simulink model "mdl_sensor_imu_16b"  (R2016b)
settings: Solver=ode4  StartTime=0.0  StopTime=20  FixedStep=0.0001  RelTol=1e-3
undefined symbols (not defined in the file): Acc_uDot_mPerScnd2, Acc_vDot_mPerScnd2, Acc_wDot_mPerScnd2, AgVel_p_radPerScnd, AgVel_q_radPerScnd, AgVel_r_radPerScnd, Par_mdlQuad
libraries: simulink x6
settings Model: Creator=Nu  LastModifiedBy=Nu

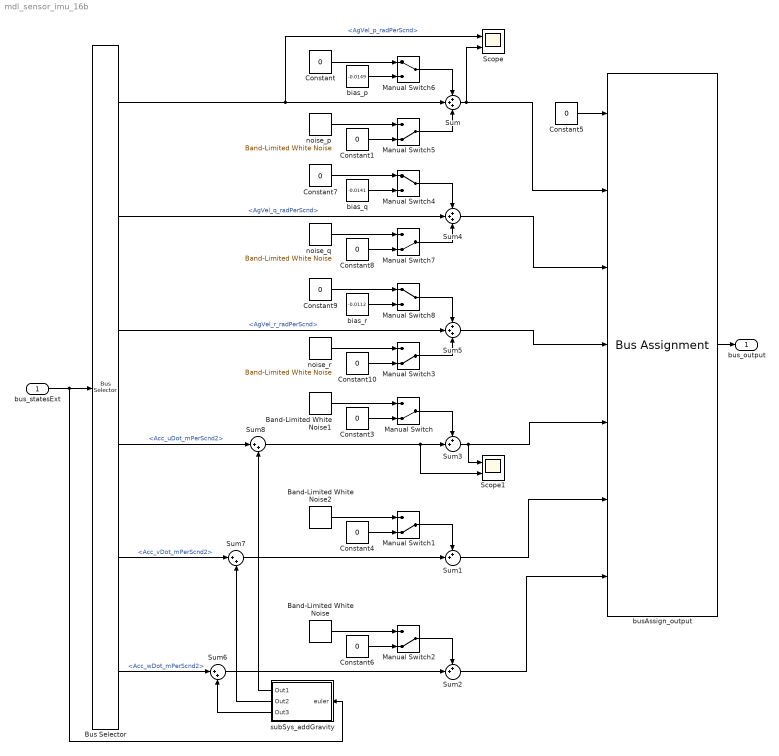
== system mdl_sensor_imu_16b ==
  bus_statesExt : Inport  OutDataTypeStr=Bus: mdl_statesExt
  Band-Limited White Noise : simulink/Sources/Band-Limited White Noise  Cov=8e-06  Ts=0.001  seed=[23341]
  Band-Limited White Noise1 : simulink/Sources/Band-Limited White Noise  Cov=8e-07  Ts=0.001  seed=[23340]
  Band-Limited White Noise2 : simulink/Sources/Band-Limited White Noise  Cov=1e-07  Ts=0.001  seed=[23311]
  Bus Selector : BusSelector  OutputSignals=AgVel_p_radPerScnd,AgVel_q_radPerScnd,AgVel_r_radPerScnd,Acc_uDot_mPerScnd2,Acc_vDot_mPerScnd2,Acc_wDot_mPerScnd2
  Constant{,1,3..4,6..10} (9 alike) : Constant  Value=0
  Constant5 : Constant  Value=0  OutDataTypeStr=Bus: mdl_output
  Manual Switch{,1..3,5,7} (6 alike) : ManualSwitch  CurrentSetting=0
  Manual Switch4 : ManualSwitch
  Manual Switch6 : ManualSwitch
  Manual Switch8 : ManualSwitch
  Scope : Scope  NumInputPorts=2
  Scope1 : Scope  NumInputPorts=2
  Sum : Sum  Inputs=+++
  Sum1 : Sum  Inputs=++|
  Sum2 : Sum  Inputs=++|
  Sum3 : Sum  Inputs=++|
  Sum4 : Sum  Inputs=+++
  Sum5 : Sum  Inputs=+++
  Sum6 : Sum  Inputs=|++
  Sum7 : Sum  Inputs=|++
  Sum8 : Sum  Inputs=|++
  bias_p : Constant  Value=-0.0149
  bias_q : Constant  Value=-0.0141
  bias_r : Constant  Value=-0.0112
  busAssign_output : BusAssignment  AssignedSignals=AgVel_p_radPerScnd,AgVel_q_radPerScnd,AgVel_r_radPerScnd,Acc_uDot_mPerScnd2,Acc_vDot_mPerScnd2,Acc_wDot_mPerScnd2
  noise_p : simulink/Sources/Band-Limited White Noise  Cov=4e-08  Ts=0.001  seed=[23340]
  noise_q : simulink/Sources/Band-Limited White Noise  Cov=4e-08  Ts=0.001  seed=[23311]
  noise_r : simulink/Sources/Band-Limited White Noise  Cov=4e-08  Ts=0.001  seed=[23341]
  subSys_addGravity : Subsystem
  bus_output : Outport  OutDataTypeStr=Bus: mdl_output
  wires:
  Sum/1 -> Scope/2, busAssign_output/2
  Sum6/1 -> Sum2/2
  Bus Selector/4 -> Sum8/1  "<Acc_uDot_mPerScnd2>"
  Bus Selector/6 -> Sum6/1  "<Acc_wDot_mPerScnd2>"
  Bus Selector/5 -> Sum7/1  "<Acc_vDot_mPerScnd2>"
  Manual Switch2/1 -> Sum2/1
  Manual Switch1/1 -> Sum1/1
  Manual Switch/1 -> Sum3/1
  bias_p/1 -> Manual Switch6/2
  noise_p/1 -> Manual Switch5/1
  bias_q/1 -> Manual Switch4/2
  noise_q/1 -> Manual Switch7/1
  Bus Selector/3 -> Sum5/2  "<AgVel_r_radPerScnd>"
  bus_statesExt/1 -> subSys_addGravity/1(euler), Bus Selector/1
  Sum2/1 -> busAssign_output/7
  Sum1/1 -> busAssign_output/6
  Sum3/1 -> busAssign_output/5, Scope1/1
  busAssign_output/1 -> bus_output/1
  Constant5/1 -> busAssign_output/1
  Bus Selector/2 -> Sum4/2  "<AgVel_q_radPerScnd>"
  Bus Selector/1 -> Scope/1, Sum/2  "<AgVel_p_radPerScnd>"
  Manual Switch6/1 -> Sum/1
  Constant/1 -> Manual Switch6/1
  Manual Switch5/1 -> Sum/3
  Constant1/1 -> Manual Switch5/2
  Constant7/1 -> Manual Switch4/1
  Manual Switch4/1 -> Sum4/1
  Constant8/1 -> Manual Switch7/2
  Manual Switch7/1 -> Sum4/3
  Sum4/1 -> busAssign_output/3
  Sum5/1 -> busAssign_output/4
  Manual Switch8/1 -> Sum5/1
  bias_r/1 -> Manual Switch8/2
  Constant9/1 -> Manual Switch8/1
  Manual Switch3/1 -> Sum5/3
  noise_r/1 -> Manual Switch3/1
  Constant10/1 -> Manual Switch3/2
  Band-Limited White Noise/1 -> Manual Switch2/1
  Constant6/1 -> Manual Switch2/2
  Constant4/1 -> Manual Switch1/2
  Band-Limited White Noise2/1 -> Manual Switch1/1
  Constant3/1 -> Manual Switch/2
  Band-Limited White Noise1/1 -> Manual Switch/1
  Sum7/1 -> Sum1/2
  Sum8/1 -> Scope1/2, Sum3/2
  subSys_addGravity/1(Out1) -> Sum8/2
  subSys_addGravity/2(Out2) -> Sum7/2
  subSys_addGravity/3(Out3) -> Sum6/2

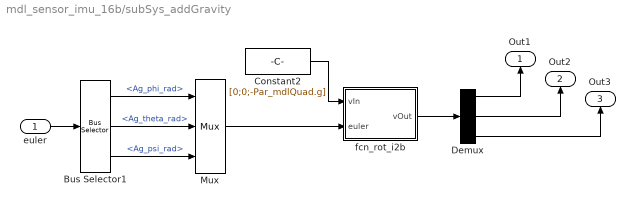
== system mdl_sensor_imu_16b/subSys_addGravity ==
  euler : Inport
  Bus Selector1 : BusSelector  OutputSignals=Ag_phi_rad,Ag_theta_rad,Ag_psi_rad
  Constant2 : Constant  Value=[0;0;-Par_mdlQuad.g]
  Demux : Demux  Outputs=3
  Mux : Mux  Inputs=3
  fcn_rot_i2b : MATLAB Function  TreatAsAtomicUnit=on
  Out1 : Outport
  Out2 : Outport  Port=2
  Out3 : Outport  Port=3
  wires:
  fcn_rot_i2b/1(vOut) -> Demux/1
  euler/1 -> Bus Selector1/1
  Bus Selector1/3 -> Mux/3  "<Ag_psi_rad>"
  Bus Selector1/2 -> Mux/2  "<Ag_theta_rad>"
  Constant2/1 -> fcn_rot_i2b/1(vIn)
  Mux/1 -> fcn_rot_i2b/2(euler)
  Bus Selector1/1 -> Mux/1  "<Ag_phi_rad>"
  Demux/1 -> Out1/1
  Demux/3 -> Out3/1
  Demux/2 -> Out2/1

== matlab function mdl_sensor_imu_16b/subSys_addGravity/fcn_rot_i2b ==
  data: vIn input; euler input; vOut output
function vOut = fcn(vIn, euler)

vOut = rot_euler(vIn, euler, 'to-body-frame');
